simulink model "allmodes"  (Simulink 7.4)
settings: Solver=ode23tb  StartTime=0.0  StopTime=inf  MaxStep=1e-4  RelTol=1e-4
undefined symbols (not defined in the file): Ion, Lithium
libraries: powerlib x185, electricdrivelib x21, powerlib_extras x19, simulink x5
(part 1 of 7)
settings Model: RequirementInfo={} %GIDa_7aa36dfb_5f63_4103_a377_470aa43c19e1  Creator=SESHNUR  LastModifiedBy=Administrator

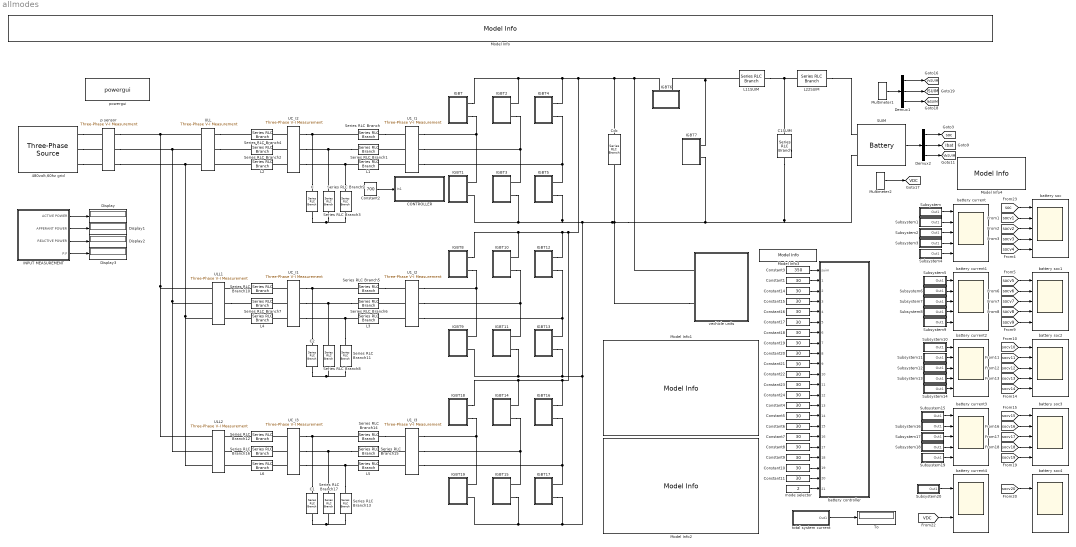
== system allmodes ==
  480volt,60hz grid : powerlib/Electrical Sources/Three-Phase Source  DialogController=POWERSYS.PowerSysDialog  SystemSampleTime=-1  Voltage=480  PhaseAngle=0  Frequency=60  InternalConnection=Yg  SpecifyImpedance=on  Resistance=0.8929  Inductance=16.58e-3  ShortCircuitLevel=50e6  BaseVoltage=400  XRratio=7
  C : powerlib/Elements/Series RLC Branch  DialogController=POWERSYS.PowerSysDialog  PhysicalDomain=powersysdomain  SubClassName=unknown  LeftPortType=p1  RightPortType=p1  LConnTagsString=__new0  RConnTagsString=__new0  BranchType=RC  Resistance=0.75  Inductance=1e-3  SetiL0=off  InitialCurrent=0  Capacitance=33e-6  Setx0=on  InitialVoltage=0  Measurements=Branch voltage and current
  C1 : powerlib/Elements/Series RLC Branch  DialogController=POWERSYS.PowerSysDialog  PhysicalDomain=powersysdomain  SubClassName=unknown  LeftPortType=p1  RightPortType=p1  LConnTagsString=__new0  RConnTagsString=__new0  BranchType=RC  Resistance=0.75  Inductance=1e-3  SetiL0=off  InitialCurrent=0  Capacitance=33e-6  Setx0=on  InitialVoltage=0  Measurements=Branch voltage and current
  C1SUIM : powerlib/Elements/Series RLC Branch  DialogController=POWERSYS.PowerSysDialog  PhysicalDomain=powersysdomain  SubClassName=unknown  LeftPortType=p1  RightPortType=p1  LConnTagsString=__new0  RConnTagsString=__new0  BranchType=C  Resistance=0.75  Inductance=1e-3  SetiL0=off  InitialCurrent=0  Capacitance=33e-6  Setx0=on  InitialVoltage=0  Measurements=Branch voltage and current
  C2 : powerlib/Elements/Series RLC Branch  DialogController=POWERSYS.PowerSysDialog  PhysicalDomain=powersysdomain  SubClassName=unknown  LeftPortType=p1  RightPortType=p1  LConnTagsString=__new0  RConnTagsString=__new0  BranchType=RC  Resistance=0.75  Inductance=1e-3  SetiL0=off  InitialCurrent=0  Capacitance=33e-6  Setx0=on  InitialVoltage=0  Measurements=Branch voltage and current
  CONTROLLER : Subsystem
  Cdc : powerlib/Elements/Series RLC Branch  DialogController=POWERSYS.PowerSysDialog  PhysicalDomain=powersysdomain  SubClassName=unknown  LeftPortType=p1  RightPortType=p1  LConnTagsString=__new0  RConnTagsString=__new0  BranchType=C  Resistance=0.002  Inductance=1e-3  SetiL0=off  InitialCurrent=0  Capacitance=0.5  Setx0=on  InitialVoltage=500  Measurements=Branch voltage and current
  Constant{1,4..11,14..24} (20 alike) : Constant  Value=30  OutDataType=fixdt(1, 16)  OutScaling=2^0
  Constant2 : Constant  Value=700  OutDataType=fixdt(1, 16)  OutScaling=2^0
  Constant3 : Constant  Value=350  OutDataType=fixdt(1, 16)  OutScaling=2^0
  Demux1 : Demux  Outputs=3
  Demux2 : Demux  Outputs=3
  Display{,1..3} (4 alike) : Display
  IGBT : Subsystem
  IGBT1 : Subsystem
  IGBT10 : Subsystem
  IGBT11 : Subsystem
  IGBT12 : Subsystem
  IGBT13 : Subsystem
  IGBT14 : Subsystem
  IGBT15 : Subsystem
  IGBT16 : Subsystem
  IGBT17 : Subsystem
  IGBT18 : Subsystem
  IGBT19 : Subsystem
  IGBT2 : Subsystem
  IGBT3 : Subsystem
  IGBT4 : Subsystem
  IGBT5 : Subsystem
  IGBT6 : Subsystem
  IGBT7 : Subsystem
  IGBT8 : Subsystem
  IGBT9 : Subsystem
  INPUT MEASUREMENT : Subsystem
  L1 : powerlib/Elements/Series RLC Branch  DialogController=POWERSYS.PowerSysDialog  PhysicalDomain=powersysdomain  SubClassName=unknown  LeftPortType=p1  RightPortType=p1  LConnTagsString=__new0  RConnTagsString=__new0  BranchType=RL  Resistance=1e-3  Inductance=5e-4  SetiL0=off  InitialCurrent=0  Capacitance=1e-6  Setx0=off  InitialVoltage=0  Measurements=Branch voltage
  L11SUIM : powerlib/Elements/Series RLC Branch  DialogController=POWERSYS.PowerSysDialog  PhysicalDomain=powersysdomain  SubClassName=unknown  LeftPortType=p1  RightPortType=p1  LConnTagsString=__new0  RConnTagsString=__new0  BranchType=RL  Resistance=1e-3  Inductance=0.0033  SetiL0=off  InitialCurrent=0  Capacitance=1e-6  Setx0=off  InitialVoltage=0  Measurements=Branch voltage and current
  L2 : powerlib/Elements/Series RLC Branch  DialogController=POWERSYS.PowerSysDialog  PhysicalDomain=powersysdomain  SubClassName=unknown  LeftPortType=p1  RightPortType=p1  LConnTagsString=__new0  RConnTagsString=__new0  BranchType=RL  Resistance=1e-3  Inductance=2.5e-4  SetiL0=off  InitialCurrent=0  Capacitance=1e-6  Setx0=off  InitialVoltage=0  Measurements=Branch voltage
  L22SUIM : powerlib/Elements/Series RLC Branch  DialogController=POWERSYS.PowerSysDialog  PhysicalDomain=powersysdomain  SubClassName=unknown  LeftPortType=p1  RightPortType=p1  LConnTagsString=__new0  RConnTagsString=__new0  BranchType=RL  Resistance=1e-3  Inductance=1.2e-4  SetiL0=off  InitialCurrent=0  Capacitance=1e-6  Setx0=off  InitialVoltage=0  Measurements=Branch current
  L3 : powerlib/Elements/Series RLC Branch  DialogController=POWERSYS.PowerSysDialog  PhysicalDomain=powersysdomain  SubClassName=unknown  LeftPortType=p1  RightPortType=p1  LConnTagsString=__new0  RConnTagsString=__new0  BranchType=RL  Resistance=1e-3  Inductance=5e-4  SetiL0=off  InitialCurrent=0  Capacitance=1e-6  Setx0=off  InitialVoltage=0  Measurements=Branch voltage
  L4 : powerlib/Elements/Series RLC Branch  DialogController=POWERSYS.PowerSysDialog  PhysicalDomain=powersysdomain  SubClassName=unknown  LeftPortType=p1  RightPortType=p1  LConnTagsString=__new0  RConnTagsString=__new0  BranchType=RL  Resistance=1e-3  Inductance=2.5e-4  SetiL0=off  InitialCurrent=0  Capacitance=1e-6  Setx0=off  InitialVoltage=0  Measurements=Branch voltage
  L5 : powerlib/Elements/Series RLC Branch  DialogController=POWERSYS.PowerSysDialog  PhysicalDomain=powersysdomain  SubClassName=unknown  LeftPortType=p1  RightPortType=p1  LConnTagsString=__new0  RConnTagsString=__new0  BranchType=RL  Resistance=1e-3  Inductance=5e-4  SetiL0=off  InitialCurrent=0  Capacitance=1e-6  Setx0=off  InitialVoltage=0  Measurements=Branch voltage
  L6 : powerlib/Elements/Series RLC Branch  DialogController=POWERSYS.PowerSysDialog  PhysicalDomain=powersysdomain  SubClassName=unknown  LeftPortType=p1  RightPortType=p1  LConnTagsString=__new0  RConnTagsString=__new0  BranchType=RL  Resistance=1e-3  Inductance=2.5e-4  SetiL0=off  InitialCurrent=0  Capacitance=1e-6  Setx0=off  InitialVoltage=0  Measurements=Branch voltage
  Model Info : simulink/Model-Wide Utilities/Model Info  SystemSampleTime=-1  InitialBlockCM=None  BlockCM=None  Frame=on  DisplayStringWithTags=BI-Directional/Centralized/fast charging system for plug-in and all electric vechicles with built-im energy storage interface and v2g and energy management system(EMS) with demand response capabilities  HorizontalTextAlignment=Center  LeftAlignmentValue=0.5  SourceBlockDiagram=allmodes  TagMaxNumber=20
  Model Info1 : simulink/Model-Wide Utilities/Model Info  SystemSampleTime=-1  InitialBlockCM=None  BlockCM=None  Frame=on  DisplayStringWithTags=|  HorizontalTextAlignment=Center  LeftAlignmentValue=0.5  SourceBlockDiagram=allmodes  TagMaxNumber=20
      | suim:
      |     ref-
      |      minimum current:-350
      |      maximum current:350
      | rating: 400v,350A
      |     charging time:
      |          i=(0.3c for trickle charge --350*0.3)
      |             (7c for fast charge --350*7)
      | -ve reference for discharge mode
      | +ve reference for charging mode
  Model Info2 : simulink/Model-Wide Utilities/Model Info  SystemSampleTime=-1  InitialBlockCM=None  BlockCM=None  Frame=on  DisplayStringWithTags=|  HorizontalTextAlignment=Center  LeftAlignmentValue=0.5  SourceBlockDiagram=allmodes  TagMaxNumber=20
      | vechicle::
      |     ref-
      |      minimum current:-30
      |      maximum current:30
      | rating: 200v,30A
      |     charging time:
      |          i=(0.3c for trickle charge --30*0.3)
      |             (7c for fast charge --30*7)
      | -ve reference for discharge mode
      | +ve reference for charging mode
  Model Info3 : simulink/Model-Wide Utilities/Model Info  SystemSampleTime=-1  InitialBlockCM=None  BlockCM=None  Frame=on  DisplayStringWithTags=reference  HorizontalTextAlignment=Left  LeftAlignmentValue=0.02  SourceBlockDiagram=allmodes  TagMaxNumber=20
  Model Info4 : simulink/Model-Wide Utilities/Model Info  SystemSampleTime=-1  InitialBlockCM=None  BlockCM=None  Frame=on  DisplayStringWithTags="yellow - reference pin-  actual"  HorizontalTextAlignment=Center  LeftAlignmentValue=0.5  SourceBlockDiagram=allmodes  TagMaxNumber=20
  Multimeter1 : powerlib/Measurements/Multimeter  SystemSampleTime=-1  PhasorSimulation=off  OutputType=Complex  sel=[3 118 119]  L=119  Gain=[1 1 1]  yselected={'Ub: C1SUIM','Ib: L11SUIM','Ib: L22SUIM'};  PSBOutputType=1  PSBequivalent=0  AxesSetting=[0,0.1,-100,100]  Display=0  SavedBlockNames=-11
  Multimeter2 : powerlib/Measurements/Multimeter  SystemSampleTime=-1  PhasorSimulation=off  OutputType=Complex  sel=45  L=119  Gain=1  yselected={'Ub: Cdc'};  PSBOutputType=1  PSBequivalent=0  AxesSetting=[0,0.1,-100,100]  Display=0  SavedBlockNames=-11
  SUIM : electricdrivelib/Extra Sources/Battery  DialogController=POWERSYS.PowerSysDialog  SystemSampleTime=-1  BatType=Lithium-Ion  ShowDetailedParameters=off  NomV=400  NomQ=350  SOC=50  PresetModel=on  MaxQ=350  FullV=465.5949  Dis_rate=152.1739  R=0.011429  Normal_OP=316.5217  expZone="[432.1543      17.19565]"  Dis_Char=off  current=[2500 1000]  Units=Ampere-hour  Batt_Tr=30
  Series RLC Branch{,1,5..6,14..15} (6 alike) : powerlib/Elements/Series RLC Branch  DialogController=POWERSYS.PowerSysDialog  PhysicalDomain=powersysdomain  SubClassName=unknown  LeftPortType=p1  RightPortType=p1  LConnTagsString=__new0  RConnTagsString=__new0  BranchType=RL  Resistance=1e-3  Inductance=5e-4  SetiL0=off  InitialCurrent=0  Capacitance=1e-6  Setx0=off  InitialVoltage=0  Measurements=None
  Series RLC Branch{2,4,7,10,12,16} (6 alike) : powerlib/Elements/Series RLC Branch  DialogController=POWERSYS.PowerSysDialog  PhysicalDomain=powersysdomain  SubClassName=unknown  LeftPortType=p1  RightPortType=p1  LConnTagsString=__new0  RConnTagsString=__new0  BranchType=RL  Resistance=1e-3  Inductance=2.5e-4  SetiL0=off  InitialCurrent=0  Capacitance=1e-6  Setx0=off  InitialVoltage=0  Measurements=None
  Series RLC Branch{3,8..9,11,13,17} (6 alike) : powerlib/Elements/Series RLC Branch  DialogController=POWERSYS.PowerSysDialog  PhysicalDomain=powersysdomain  SubClassName=unknown  LeftPortType=p1  RightPortType=p1  LConnTagsString=__new0  RConnTagsString=__new0  BranchType=RC  Resistance=0.75  Inductance=1e-3  SetiL0=off  InitialCurrent=0  Capacitance=33e-6  Setx0=on  InitialVoltage=0  Measurements=None
  Subsystem : Subsystem
  Subsystem1 : Subsystem
  Subsystem10 : Subsystem
  Subsystem11 : Subsystem
  Subsystem12 : Subsystem
  Subsystem13 : Subsystem
  Subsystem14 : Subsystem
  Subsystem15 : Subsystem
  Subsystem16 : Subsystem
  Subsystem17 : Subsystem
  Subsystem18 : Subsystem
  Subsystem19 : Subsystem
  Subsystem2 : Subsystem
  Subsystem20 : Subsystem
  Subsystem3 : Subsystem
  Subsystem4 : Subsystem
  Subsystem5 : Subsystem
  Subsystem6 : Subsystem
  Subsystem7 : Subsystem
  Subsystem8 : Subsystem
  Subsystem9 : Subsystem
  To : Display
  U1_I1 : powerlib/Measurements/Three-Phase V-I Measurement  DialogController=POWERSYS.PowerSysDialog  SystemSampleTime=-1  VoltageMeasurement=phase-to-phase  SetLabelV=on  LabelV=U1  Vpu=off  CurrentMeasurement=yes  SetLabelI=on  LabelI=I1  Ipu=off  Pbase=100e6  Vbase=500e3  OutputType=Complex  PhasorSimulation=off  PSBequivalent=0
  U1_I2 : powerlib/Measurements/Three-Phase V-I Measurement  DialogController=POWERSYS.PowerSysDialog  SystemSampleTime=-1  VoltageMeasurement=phase-to-phase  SetLabelV=on  LabelV=U11  Vpu=off  CurrentMeasurement=yes  SetLabelI=on  LabelI=I11  Ipu=off  Pbase=100e6  Vbase=500e3  OutputType=Complex  PhasorSimulation=off  PSBequivalent=0
  U1_I3 : powerlib/Measurements/Three-Phase V-I Measurement  DialogController=POWERSYS.PowerSysDialog  SystemSampleTime=-1  VoltageMeasurement=phase-to-phase  SetLabelV=on  LabelV=U111  Vpu=off  CurrentMeasurement=yes  SetLabelI=on  LabelI=I111  Ipu=off  Pbase=100e6  Vbase=500e3  OutputType=Complex  PhasorSimulation=off  PSBequivalent=0
  UC_I1 : powerlib/Measurements/Three-Phase V-I Measurement  DialogController=POWERSYS.PowerSysDialog  SystemSampleTime=-1  VoltageMeasurement=phase-to-ground  SetLabelV=on  LabelV=Uc1  Vpu=off  CurrentMeasurement=yes  SetLabelI=on  LabelI=I21  Ipu=off  Pbase=100e6  Vbase=500e3  OutputType=Complex  PhasorSimulation=off  PSBequivalent=0
  UC_I2 : powerlib/Measurements/Three-Phase V-I Measurement  DialogController=POWERSYS.PowerSysDialog  SystemSampleTime=-1  VoltageMeasurement=phase-to-ground  SetLabelV=on  LabelV=Uc  Vpu=off  CurrentMeasurement=yes  SetLabelI=on  LabelI=I2  Ipu=off  Pbase=100e6  Vbase=500e3  OutputType=Complex  PhasorSimulation=off  PSBequivalent=0
  UC_I3 : powerlib/Measurements/Three-Phase V-I Measurement  DialogController=POWERSYS.PowerSysDialog  SystemSampleTime=-1  VoltageMeasurement=phase-to-ground  SetLabelV=on  LabelV=Uc11  Vpu=off  CurrentMeasurement=yes  SetLabelI=on  LabelI=I211  Ipu=off  Pbase=100e6  Vbase=500e3  OutputType=Complex  PhasorSimulation=off  PSBequivalent=0
  ULL : powerlib/Measurements/Three-Phase V-I Measurement  DialogController=POWERSYS.PowerSysDialog  SystemSampleTime=-1  VoltageMeasurement=phase-to-ground  SetLabelV=on  LabelV=ULL  Vpu=off  CurrentMeasurement=yes  SetLabelI=on  LabelI=IL  Ipu=off  Pbase=100e6  Vbase=500e3  OutputType=Complex  PhasorSimulation=off  PSBequivalent=0
  ULL1 : powerlib/Measurements/Three-Phase V-I Measurement  DialogController=POWERSYS.PowerSysDialog  SystemSampleTime=-1  VoltageMeasurement=phase-to-ground  SetLabelV=on  LabelV=ULL1  Vpu=off  CurrentMeasurement=yes  SetLabelI=on  LabelI=IL1  Ipu=off  Pbase=100e6  Vbase=500e3  OutputType=Complex  PhasorSimulation=off  PSBequivalent=0
  ULL2 : powerlib/Measurements/Three-Phase V-I Measurement  DialogController=POWERSYS.PowerSysDialog  SystemSampleTime=-1  VoltageMeasurement=phase-to-ground  SetLabelV=on  LabelV=ULL11  Vpu=off  CurrentMeasurement=yes  SetLabelI=on  LabelI=IL11  Ipu=off  Pbase=100e6  Vbase=500e3  OutputType=Complex  PhasorSimulation=off  PSBequivalent=0
  "battery controller " : Subsystem
  battery current{,1..3} (4 alike) : Scope  NumInputPorts=5
      battery current settings: TimeRange=0.25  YMin=-250~202~195~0~0  YMax=2500~214~215~225~225  MaxDataPoints=50000  SampleInput=on  SampleTime=0.001
      battery current1 settings: TimeRange=0.25  YMin=0~0~0~0~0  YMax=225~225~225~225~225  MaxDataPoints=50000  SampleInput=on  SampleTime=0.001
      battery current2 settings: TimeRange=0.25  YMin=115~115~115~115~115  YMax=135~135~135~135~135  SaveName=ScopeData2  MaxDataPoints=50000  SampleInput=on  SampleTime=0.001
      battery current3 settings: TimeRange=0.25  YMin=189~189~189~189~189  YMax=196~196~196~196~196  SaveName=ScopeData4  MaxDataPoints=50000  SampleInput=on  SampleTime=0.001
  battery current4 : Scope  NumInputPorts=2
      settings: TimeRange=0.7000000000000001  YMin=0~706.475  YMax=210~706.75  SaveName=ScopeData5  MaxDataPoints=50000  SampleInput=on  SampleTime=0.001
  battery soc{,1..3} (4 alike) : Scope  NumInputPorts=5
      battery soc settings: TimeRange=0.25  YMin=50~10.487~50.487~50~50  YMax=50~10.4893~50.4893~50~50  SaveName=ScopeData3  MaxDataPoints=50000  SampleInput=on  SampleTime=0.001
      battery soc1 settings: TimeRange=0.25  YMin=2.00683~50.0074~50.0074~50.0074~50.0074  YMax=2.00707~50.0076~50.0076~50.0076~50.0076  SaveName=ScopeData6  MaxDataPoints=50000  SampleInput=on  SampleTime=0.001
      battery soc2 settings: TimeRange=0.25  YMin=0.0026805~0.0026805~0.0026805~0.0026805~0.0026805  YMax=0.0026845~0.0026845~0.0026845~0.0026845~0.0026845  SaveName=ScopeData8  MaxDataPoints=50000  SampleInput=on  SampleTime=0.001
      battery soc3 settings: TimeRange=0.25  YMin=0~0~0~0~0  YMax=130~130~130~130~130  SaveName=ScopeData9  MaxDataPoints=50000  SampleInput=on  SampleTime=0.001
  battery soc4 : Scope  NumInputPorts=2
      settings: TimeRange=0.25  YMin=47.5~-1  YMax=52.5~1  SaveName=ScopeData10  MaxDataPoints=50000  SampleInput=on  SampleTime=0.001
  mode selector : Constant  Value=2  OutDataType=fixdt(1, 16)  OutScaling=2^0
  p sensor : powerlib/Measurements/Three-Phase V-I Measurement  DialogController=POWERSYS.PowerSysDialog  SystemSampleTime=-1  VoltageMeasurement=phase-to-ground  SetLabelV=on  LabelV=VIN  Vpu=off  CurrentMeasurement=yes  SetLabelI=on  LabelI=IIN  Ipu=off  Pbase=100e6  Vbase=500e3  OutputType=Complex  PhasorSimulation=off  PSBequivalent=0
  powergui : powerlib/powergui  Priority=1  SystemSampleTime=-1  SimulationMode=Discrete  SampleTime=50e-6  frequency=60  SPID=off  DisableSnubberDevices=off  DisableRonSwitches=off  DisableVfSwitches=off  SwTol=0  Interpol=off  frequencyindice=60  echomessages=off  HookPort=off  DisplayEquations=off  FunctionMessages=off  EnableUseOfTLC=off  x0status=blocks  RestoreLinks=warning  Frange=[0:2:500]  Ylog=off  Xlog=on  ShowGrid=off  save=off  variable=ZData  ZoomFFT=on  StartTime=0.0  cycles=1  DisplayStyle=1  fundamental=60  FreqAxis=off  MaxFrequency=1000  frequencyindicesteady=1  RmsSteady=1  display=off  Ts=0  methode=off
  total system current : Subsystem
  vechicle units : Subsystem
  tag scope: ISUIM=global, IbSUIM=global, Ibat=global, VDC=global, VbSUIM=global, VcSUIM=global, soc=global
  wires:
  SUIM/1 -> Demux2/1
  Demux2/1 -> [soc]
  Demux2/2 -> [Ibat]
  Demux2/3 -> [VbSUIM]
  Multimeter1/1 -> Demux1/1
  INPUT MEASUREMENT/1(ACTIVE POWER) -> Display/1
  INPUT MEASUREMENT/2(APPERANT POWER) -> Display1/1
  INPUT MEASUREMENT/3(REACTIVE POWER) -> Display2/1
  INPUT MEASUREMENT/4(P.F) -> Display3/1
  Demux1/2 -> [ISUIM]
  Demux1/3 -> [IbSUIM]
  Demux1/1 -> [VcSUIM]
  Constant2/1 -> CONTROLLER/1(In1)
  Constant3/1 -> "battery controller "/1(suim)
  Constant1/1 -> "battery controller "/2(1)
  Constant14/1 -> "battery controller "/3(2)
  Constant15/1 -> "battery controller "/4(3)
  Constant16/1 -> "battery controller "/5(4)
  Constant17/1 -> "battery controller "/6(5)
  Constant18/1 -> "battery controller "/7(6)
  Constant19/1 -> "battery controller "/8(7)
  Constant20/1 -> "battery controller "/9(8)
  Constant21/1 -> "battery controller "/10(9)
  Constant22/1 -> "battery controller "/11(10)
  Constant23/1 -> "battery controller "/12(11)
  Constant24/1 -> "battery controller "/13(12)
  Constant4/1 -> "battery controller "/14(13)
  Constant5/1 -> "battery controller "/15(14)
  Constant6/1 -> "battery controller "/16(15)
  Constant7/1 -> "battery controller "/17(16)
  Constant8/1 -> "battery controller "/18(17)
  Constant9/1 -> "battery controller "/19(18)
  Constant10/1 -> "battery controller "/20(19)
  Constant11/1 -> "battery controller "/21(20)
  mode selector/1 -> "battery controller "/22(21)
  Multimeter2/1 -> [VDC]
  [VDC] -> battery current4/2
  Subsystem/1(Out1) -> battery current/1
  Subsystem1/1(Out1) -> battery current/2
  Subsystem2/1(Out1) -> battery current/3
  Subsystem3/1(Out1) -> battery current/4
  Subsystem4/1(Out1) -> battery current/5
  Subsystem5/1(Out1) -> battery current1/1
  Subsystem6/1(Out1) -> battery current1/2
  Subsystem7/1(Out1) -> battery current1/3
  Subsystem8/1(Out1) -> battery current1/4
  Subsystem9/1(Out1) -> battery current1/5
  Subsystem10/1(Out1) -> battery current2/1
  Subsystem11/1(Out1) -> battery current2/2
  Subsystem12/1(Out1) -> battery current2/3
  Subsystem13/1(Out1) -> battery current2/4
  Subsystem14/1(Out1) -> battery current2/5
  Subsystem15/1(Out1) -> battery current3/1
  Subsystem16/1(Out1) -> battery current3/2
  Subsystem17/1(Out1) -> battery current3/3
  Subsystem18/1(Out1) -> battery current3/4
  Subsystem19/1(Out1) -> battery current3/5
  Subsystem20/1(Out1) -> battery current4/1
  total system current/1(Out1) -> To/1
  [soc] -> battery soc/1
  [socv1] -> battery soc/2
  [socv2] -> battery soc/3
  [socv3] -> battery soc/4
  [socv4] -> battery soc/5
  [socv5] -> battery soc1/1
  [socv6] -> battery soc1/2
  [socv7] -> battery soc1/3
  [socv8] -> battery soc1/4
  [socv9] -> battery soc1/5
  [socv10] -> battery soc2/1
  [socv11] -> battery soc2/2
  [socv12] -> battery soc2/3
  [socv13] -> battery soc2/4
  [socv14] -> battery soc2/5
  [socv15] -> battery soc3/1
  [socv16] -> battery soc3/2
  [socv17] -> battery soc3/3
  [socv18] -> battery soc3/4
  [socv19] -> battery soc3/5
  [socv20] -> battery soc4/1
  connections:
  Series RLC Branch1/LConn1 -- Series RLC Branch3/LConn1 -- UC_I2/RConn2
  C/LConn1 -- UC_I2/RConn1 -- Series RLC Branch/LConn1
  Series RLC Branch9/LConn1 -- UC_I2/RConn3 -- L1/LConn1
  Series RLC Branch3/RConn1 -- C/RConn1 -- Series RLC Branch9/RConn1
  UC_I2/LConn3 -- L2/RConn1
  Series RLC Branch/RConn1 -- U1_I1/LConn1
  U1_I1/LConn3 -- L1/RConn1
  L2/LConn1 -- ULL/RConn3
  UC_I2/LConn2 -- Series RLC Branch2/RConn1
  UC_I2/LConn1 -- Series RLC Branch4/RConn1
  U1_I1/LConn2 -- Series RLC Branch1/RConn1
  ULL/RConn2 -- Series RLC Branch2/LConn1
  ULL/RConn1 -- Series RLC Branch4/LConn1
  IGBT/RConn2 -- IGBT1/RConn1 -- U1_I1/RConn1
  IGBT2/RConn2 -- IGBT3/RConn1 -- U1_I1/RConn2
  IGBT7/RConn1 -- IGBT6/RConn2 -- L11SUIM/LConn1
  IGBT4/RConn2 -- IGBT5/RConn1 -- U1_I1/RConn3
  L11SUIM/RConn1 -- L22SUIM/LConn1 -- C1SUIM/LConn1
  L22SUIM/RConn1 -- SUIM/LConn1
  Series RLC Branch6/LConn1 -- UC_I1/RConn2 -- Series RLC Branch8/LConn1
  C2/LConn1 -- Series RLC Branch5/LConn1 -- UC_I1/RConn1
  Series RLC Branch11/LConn1 -- L3/LConn1 -- UC_I1/RConn3
  Series RLC Branch8/RConn1 -- Series RLC Branch11/RConn1 -- C2/RConn1
  IGBT8/RConn2 -- U1_I2/RConn1 -- IGBT9/RConn1
  IGBT10/RConn2 -- U1_I2/RConn2 -- IGBT11/RConn1
  IGBT12/RConn2 -- U1_I2/RConn3 -- IGBT13/RConn1
  L4/LConn1 -- ULL1/RConn3
  ULL1/RConn1 -- Series RLC Branch10/LConn1
  U1_I2/LConn2 -- Series RLC Branch6/RConn1
  UC_I1/LConn3 -- L4/RConn1
  ULL1/RConn2 -- Series RLC Branch7/LConn1
  U1_I2/LConn3 -- L3/RConn1
  Series RLC Branch5/RConn1 -- U1_I2/LConn1
  UC_I1/LConn2 -- Series RLC Branch7/RConn1
  UC_I1/LConn1 -- Series RLC Branch10/RConn1
  480volt,60hz grid/RConn1 -- p sensor/LConn1
  480volt,60hz grid/RConn2 -- p sensor/LConn2
  480volt,60hz grid/RConn3 -- p sensor/LConn3
  p sensor/RConn3 -- ULL/LConn3 -- ULL1/LConn3 -- ULL2/LConn3
  p sensor/RConn2 -- ULL/LConn2 -- ULL1/LConn2 -- ULL2/LConn2
  p sensor/RConn1 -- ULL/LConn1 -- ULL1/LConn1 -- ULL2/LConn1
  Series RLC Branch15/LConn1 -- Series RLC Branch17/LConn1 -- UC_I3/RConn2
  C1/LConn1 -- UC_I3/RConn1 -- Series RLC Branch14/LConn1
  Series RLC Branch13/LConn1 -- UC_I3/RConn3 -- L5/LConn1
  Series RLC Branch17/RConn1 -- C1/RConn1 -- Series RLC Branch13/RConn1
  IGBT18/RConn2 -- IGBT19/RConn1 -- U1_I3/RConn1
  IGBT14/RConn2 -- IGBT15/RConn1 -- U1_I3/RConn2
  IGBT16/RConn2 -- IGBT17/RConn1 -- U1_I3/RConn3
  ULL2/RConn1 -- Series RLC Branch12/LConn1
  U1_I3/LConn2 -- Series RLC Branch15/RConn1
  ULL2/RConn2 -- Series RLC Branch16/LConn1
  UC_I3/LConn3 -- L6/RConn1
  L6/LConn1 -- ULL2/RConn3
  UC_I3/LConn2 -- Series RLC Branch16/RConn1
  U1_I3/LConn3 -- L5/RConn1
  UC_I3/LConn1 -- Series RLC Branch12/RConn1
  Series RLC Branch14/RConn1 -- U1_I3/LConn1
  vechicle units/LConn1 -- IGBT6/RConn1 -- IGBT12/RConn1 -- IGBT10/RConn1 -- IGBT8/RConn1 -- IGBT16/RConn1 -- IGBT18/RConn1 -- IGBT14/RConn1 -- IGBT4/RConn1 -- IGBT/RConn1 -- IGBT2/RConn1 -- Cdc/LConn1
  vechicle units/LConn2 -- IGBT17/RConn2 -- IGBT15/RConn2 -- IGBT19/RConn2 -- IGBT13/RConn2 -- IGBT9/RConn2 -- IGBT11/RConn2 -- IGBT5/RConn2 -- IGBT3/RConn2 -- IGBT1/RConn2 -- C1SUIM/RConn1 -- SUIM/LConn2 -- IGBT7/RConn2 -- Cdc/RConn1

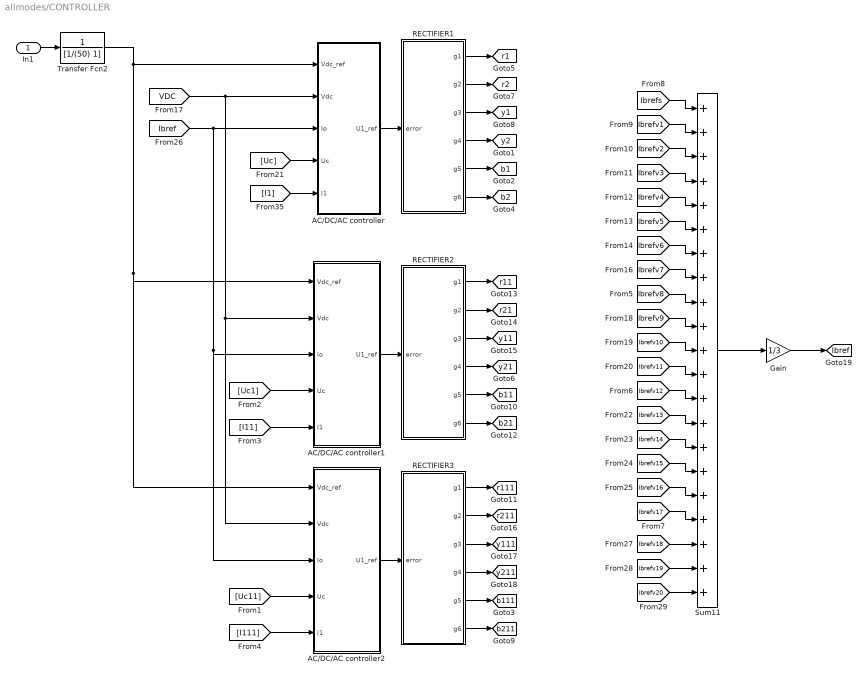
== system allmodes/CONTROLLER ==
  In1 : Inport
  AC/DC/AC controller : Subsystem
  AC/DC/AC controller1 : Subsystem
  AC/DC/AC controller2 : Subsystem
  Gain : Gain  Gain=1/3  ParameterDataType=fixdt(1, 16)  ParameterScaling=2^0  OutDataType=fixdt(1, 16)  OutScaling=2^0
  RECTIFIER1 : Subsystem  mask{fsw=5e3}
      mask prompts: fsw "switching frequency"
  RECTIFIER2 : Subsystem  mask{fsw=5e3}
      mask prompts: fsw "switching frequency"
  RECTIFIER3 : Subsystem  mask{fsw=5e3}
      mask prompts: fsw "switching frequency"
  Sum11 : Sum  Inputs=+++++++++++++++++++++  OutDataType=fixdt(1, 16)  OutScaling=2^0
  Transfer Fcn2 : TransferFcn  Numerator=1  Denominator=[1/(50) 1]
  tag scope: Ibref=global, b111=global, b11=global, b1=global, b211=global, b21=global, b2=global, r111=global, r11=global, r1=global, r211=global, r21=global, r2=global, y111=global, y11=global, y1=global, y211=global, y21=global, y2=global
  wires:
  RECTIFIER1/1(g1) -> [r1]
  RECTIFIER1/2(g2) -> [r2]
  RECTIFIER1/3(g3) -> [y1]
  RECTIFIER1/4(g4) -> [y2]
  RECTIFIER1/5(g5) -> [b1]
  RECTIFIER1/6(g6) -> [b2]
  RECTIFIER2/1(g1) -> [r11]
  RECTIFIER2/2(g2) -> [r21]
  RECTIFIER2/3(g3) -> [y11]
  RECTIFIER2/4(g4) -> [y21]
  RECTIFIER2/5(g5) -> [b11]
  RECTIFIER2/6(g6) -> [b21]
  [VDC] -> AC/DC/AC controller/2(Vdc), AC/DC/AC controller1/2(Vdc), AC/DC/AC controller2/2(Vdc)
  [Uc] -> AC/DC/AC controller/4(Uc)
  [I1] -> AC/DC/AC controller/5(I1)
  [Ibref] -> AC/DC/AC controller/3(Io), AC/DC/AC controller1/3(Io), AC/DC/AC controller2/3(Io)
  [Uc1] -> AC/DC/AC controller1/4(Uc)
  [I11] -> AC/DC/AC controller1/5(I1)
  AC/DC/AC controller/1(U1_ref) -> RECTIFIER1/1(error)
  AC/DC/AC controller1/1(U1_ref) -> RECTIFIER2/1(error)
  In1/1 -> Transfer Fcn2/1
  Transfer Fcn2/1 -> AC/DC/AC controller/1(Vdc_ref), AC/DC/AC controller1/1(Vdc_ref), AC/DC/AC controller2/1(Vdc_ref)
  RECTIFIER3/1(g1) -> [r111]
  RECTIFIER3/2(g2) -> [r211]
  RECTIFIER3/3(g3) -> [y111]
  RECTIFIER3/4(g4) -> [y211]
  RECTIFIER3/5(g5) -> [b111]
  RECTIFIER3/6(g6) -> [b211]
  [Uc11] -> AC/DC/AC controller2/4(Uc)
  [I111] -> AC/DC/AC controller2/5(I1)
  AC/DC/AC controller2/1(U1_ref) -> RECTIFIER3/1(error)
  [Ibrefs] -> Sum11/1
  [Ibrefv1] -> Sum11/2
  [Ibrefv2] -> Sum11/3
  [Ibrefv3] -> Sum11/4
  [Ibrefv4] -> Sum11/5
  [Ibrefv5] -> Sum11/6
  [Ibrefv6] -> Sum11/7
  [Ibrefv7] -> Sum11/8
  [Ibrefv8] -> Sum11/9
  [Ibrefv9] -> Sum11/10
  [Ibrefv10] -> Sum11/11
  [Ibrefv11] -> Sum11/12
  [Ibrefv12] -> Sum11/13
  [Ibrefv13] -> Sum11/14
  [Ibrefv14] -> Sum11/15
  [Ibrefv15] -> Sum11/16
  [Ibrefv16] -> Sum11/17
  [Ibrefv17] -> Sum11/18
  [Ibrefv18] -> Sum11/19
  [Ibrefv19] -> Sum11/20
  [Ibrefv20] -> Sum11/21
  Sum11/1 -> Gain/1
  Gain/1 -> [Ibref]

== system allmodes/IGBT ==
  IGBT/Diode : powerlib/Power Electronics/IGBT//Diode  DialogController=POWERSYS.PowerSysDialog  SystemSampleTime=-1  Ron=1e-3  Rs=1e5  Cs=inf  Measurements=off
  collector : PMIOPort  Port=1  Side=Right
  emitter : PMIOPort  Port=2  Side=Right
  wires:
  [r1] -> IGBT/Diode/1
  connections:
  collector/RConn1 -- IGBT/Diode/LConn1
  emitter/RConn1 -- IGBT/Diode/RConn1

== system allmodes/IGBT1 ==
  IGBT/Diode : powerlib/Power Electronics/IGBT//Diode  DialogController=POWERSYS.PowerSysDialog  SystemSampleTime=-1  Ron=1e-3  Rs=1e5  Cs=inf  Measurements=off
  collector : PMIOPort  Port=1  Side=Right
  emitter : PMIOPort  Port=2  Side=Right
  wires:
  [r2] -> IGBT/Diode/1
  connections:
  emitter/RConn1 -- IGBT/Diode/RConn1
  collector/RConn1 -- IGBT/Diode/LConn1

== system allmodes/IGBT10 ==
  IGBT/Diode : powerlib/Power Electronics/IGBT//Diode  DialogController=POWERSYS.PowerSysDialog  SystemSampleTime=-1  Ron=1e-3  Rs=1e5  Cs=inf  Measurements=off
  collector : PMIOPort  Port=1  Side=Right
  emitter : PMIOPort  Port=2  Side=Right
  wires:
  [y11] -> IGBT/Diode/1
  connections:
  collector/RConn1 -- IGBT/Diode/LConn1
  emitter/RConn1 -- IGBT/Diode/RConn1

== system allmodes/IGBT11 ==
  IGBT/Diode : powerlib/Power Electronics/IGBT//Diode  DialogController=POWERSYS.PowerSysDialog  SystemSampleTime=-1  Ron=1e-3  Rs=1e5  Cs=inf  Measurements=off
  collector : PMIOPort  Port=1  Side=Right
  emitter : PMIOPort  Port=2  Side=Right
  wires:
  [y21] -> IGBT/Diode/1
  connections:
  emitter/RConn1 -- IGBT/Diode/RConn1
  collector/RConn1 -- IGBT/Diode/LConn1

== system allmodes/IGBT12 ==
  IGBT/Diode : powerlib/Power Electronics/IGBT//Diode  DialogController=POWERSYS.PowerSysDialog  SystemSampleTime=-1  Ron=1e-3  Rs=1e5  Cs=inf  Measurements=off
  collector : PMIOPort  Port=1  Side=Right
  emitter : PMIOPort  Port=2  Side=Right
  wires:
  [b11] -> IGBT/Diode/1
  connections:
  emitter/RConn1 -- IGBT/Diode/RConn1
  collector/RConn1 -- IGBT/Diode/LConn1

== system allmodes/IGBT13 ==
  IGBT/Diode : powerlib/Power Electronics/IGBT//Diode  DialogController=POWERSYS.PowerSysDialog  SystemSampleTime=-1  Ron=1e-3  Rs=1e5  Cs=inf  Measurements=off
  collector : PMIOPort  Port=1  Side=Right
  emitter : PMIOPort  Port=2  Side=Right
  wires:
  [b21] -> IGBT/Diode/1
  connections:
  collector/RConn1 -- IGBT/Diode/LConn1
  emitter/RConn1 -- IGBT/Diode/RConn1

== system allmodes/IGBT14 ==
  IGBT/Diode : powerlib/Power Electronics/IGBT//Diode  DialogController=POWERSYS.PowerSysDialog  SystemSampleTime=-1  Ron=1e-3  Rs=1e5  Cs=inf  Measurements=off
  collector : PMIOPort  Port=1  Side=Right
  emitter : PMIOPort  Port=2  Side=Right
  wires:
  [y111] -> IGBT/Diode/1
  connections:
  emitter/RConn1 -- IGBT/Diode/RConn1
  collector/RConn1 -- IGBT/Diode/LConn1

== system allmodes/IGBT15 ==
  IGBT/Diode : powerlib/Power Electronics/IGBT//Diode  DialogController=POWERSYS.PowerSysDialog  SystemSampleTime=-1  Ron=1e-3  Rs=1e5  Cs=inf  Measurements=off
  collector : PMIOPort  Port=1  Side=Right
  emitter : PMIOPort  Port=2  Side=Right
  wires:
  [y211] -> IGBT/Diode/1
  connections:
  collector/RConn1 -- IGBT/Diode/LConn1
  emitter/RConn1 -- IGBT/Diode/RConn1

== system allmodes/IGBT16 ==
  IGBT/Diode : powerlib/Power Electronics/IGBT//Diode  DialogController=POWERSYS.PowerSysDialog  SystemSampleTime=-1  Ron=1e-3  Rs=1e5  Cs=inf  Measurements=off
  collector : PMIOPort  Port=1  Side=Right
  emitter : PMIOPort  Port=2  Side=Right
  wires:
  [b111] -> IGBT/Diode/1
  connections:
  collector/RConn1 -- IGBT/Diode/LConn1
  emitter/RConn1 -- IGBT/Diode/RConn1

== system allmodes/IGBT17 ==
  IGBT/Diode : powerlib/Power Electronics/IGBT//Diode  DialogController=POWERSYS.PowerSysDialog  SystemSampleTime=-1  Ron=1e-3  Rs=1e5  Cs=inf  Measurements=off
  collector : PMIOPort  Port=1  Side=Right
  emitter : PMIOPort  Port=2  Side=Right
  wires:
  [b211] -> IGBT/Diode/1
  connections:
  emitter/RConn1 -- IGBT/Diode/RConn1
  collector/RConn1 -- IGBT/Diode/LConn1

== system allmodes/IGBT18 ==
  IGBT/Diode : powerlib/Power Electronics/IGBT//Diode  DialogController=POWERSYS.PowerSysDialog  SystemSampleTime=-1  Ron=1e-3  Rs=1e5  Cs=inf  Measurements=off
  collector : PMIOPort  Port=1  Side=Right
  emitter : PMIOPort  Port=2  Side=Right
  wires:
  [r111] -> IGBT/Diode/1
  connections:
  collector/RConn1 -- IGBT/Diode/LConn1
  emitter/RConn1 -- IGBT/Diode/RConn1

== system allmodes/IGBT19 ==
  IGBT/Diode : powerlib/Power Electronics/IGBT//Diode  DialogController=POWERSYS.PowerSysDialog  SystemSampleTime=-1  Ron=1e-3  Rs=1e5  Cs=inf  Measurements=off
  collector : PMIOPort  Port=1  Side=Right
  emitter : PMIOPort  Port=2  Side=Right
  wires:
  [r211] -> IGBT/Diode/1
  connections:
  emitter/RConn1 -- IGBT/Diode/RConn1
  collector/RConn1 -- IGBT/Diode/LConn1

== system allmodes/IGBT2 ==
  IGBT/Diode : powerlib/Power Electronics/IGBT//Diode  DialogController=POWERSYS.PowerSysDialog  SystemSampleTime=-1  Ron=1e-3  Rs=1e5  Cs=inf  Measurements=off
  collector : PMIOPort  Port=1  Side=Right
  emitter : PMIOPort  Port=2  Side=Right
  wires:
  [y1] -> IGBT/Diode/1
  connections:
  emitter/RConn1 -- IGBT/Diode/RConn1
  collector/RConn1 -- IGBT/Diode/LConn1

== system allmodes/IGBT3 ==
  IGBT/Diode : powerlib/Power Electronics/IGBT//Diode  DialogController=POWERSYS.PowerSysDialog  SystemSampleTime=-1  Ron=1e-3  Rs=1e5  Cs=inf  Measurements=off
  collector : PMIOPort  Port=1  Side=Right
  emitter : PMIOPort  Port=2  Side=Right
  wires:
  [y2] -> IGBT/Diode/1
  connections:
  collector/RConn1 -- IGBT/Diode/LConn1
  emitter/RConn1 -- IGBT/Diode/RConn1

== system allmodes/IGBT4 ==
  IGBT/Diode : powerlib/Power Electronics/IGBT//Diode  DialogController=POWERSYS.PowerSysDialog  SystemSampleTime=-1  Ron=1e-3  Rs=1e5  Cs=inf  Measurements=off
  collector : PMIOPort  Port=1  Side=Right
  emitter : PMIOPort  Port=2  Side=Right
  wires:
  [b1] -> IGBT/Diode/1
  connections:
  collector/RConn1 -- IGBT/Diode/LConn1
  emitter/RConn1 -- IGBT/Diode/RConn1

== system allmodes/IGBT5 ==
  IGBT/Diode : powerlib/Power Electronics/IGBT//Diode  DialogController=POWERSYS.PowerSysDialog  SystemSampleTime=-1  Ron=1e-3  Rs=1e5  Cs=inf  Measurements=off
  collector : PMIOPort  Port=1  Side=Right
  emitter : PMIOPort  Port=2  Side=Right
  wires:
  [b2] -> IGBT/Diode/1
  connections:
  emitter/RConn1 -- IGBT/Diode/RConn1
  collector/RConn1 -- IGBT/Diode/LConn1

== system allmodes/IGBT6 ==
  IGBT/Diode : powerlib/Power Electronics/IGBT//Diode  DialogController=POWERSYS.PowerSysDialog  SystemSampleTime=-1  Ron=1e-3  Rs=1e5  Cs=inf  Measurements=off
  collector : PMIOPort  Port=1  Side=Right
  emitter : PMIOPort  Port=2  Side=Right
  wires:
  [buck] -> IGBT/Diode/1
  connections:
  emitter/RConn1 -- IGBT/Diode/RConn1
  collector/RConn1 -- IGBT/Diode/LConn1

== system allmodes/IGBT7 ==
  IGBT/Diode : powerlib/Power Electronics/IGBT//Diode  DialogController=POWERSYS.PowerSysDialog  SystemSampleTime=-1  Ron=1e-3  Rs=1e5  Cs=inf  Measurements=off
  collector : PMIOPort  Port=1  Side=Right
  emitter : PMIOPort  Port=2  Side=Right
  wires:
  [boost] -> IGBT/Diode/1
  connections:
  collector/RConn1 -- IGBT/Diode/LConn1
  emitter/RConn1 -- IGBT/Diode/RConn1

== system allmodes/IGBT8 ==
  IGBT/Diode : powerlib/Power Electronics/IGBT//Diode  DialogController=POWERSYS.PowerSysDialog  SystemSampleTime=-1  Ron=1e-3  Rs=1e5  Cs=inf  Measurements=off
  collector : PMIOPort  Port=1  Side=Right
  emitter : PMIOPort  Port=2  Side=Right
  wires:
  [r11] -> IGBT/Diode/1
  connections:
  emitter/RConn1 -- IGBT/Diode/RConn1
  collector/RConn1 -- IGBT/Diode/LConn1

== system allmodes/IGBT9 ==
  IGBT/Diode : powerlib/Power Electronics/IGBT//Diode  DialogController=POWERSYS.PowerSysDialog  SystemSampleTime=-1  Ron=1e-3  Rs=1e5  Cs=inf  Measurements=off
  collector : PMIOPort  Port=1  Side=Right
  emitter : PMIOPort  Port=2  Side=Right
  wires:
  [r21] -> IGBT/Diode/1
  connections:
  collector/RConn1 -- IGBT/Diode/LConn1
  emitter/RConn1 -- IGBT/Diode/RConn1

== system allmodes/INPUT MEASUREMENT ==
  3-phase  Instantaneous  Active & Reactive Power : powerlib_extras/Measurements/3-phase  Instantaneous  Active & Reactive Power  DialogController=POWERSYS.PowerSysDialog  SystemSampleTime=-1
  Add : Sum  OutDataType=fixdt(1, 16)  OutScaling=2^-10
  Demux : Demux  Outputs=2
  Divide : Product  Inputs=*/  OutDataType=fixdt(1, 16)  OutScaling=2^-10
  Fcn : Fcn  Expr=u(1)*u(1)
  Fcn1 : Fcn  Expr=u(1)*u(1)
  Math Function : Math  Operator=sqrt  OutDataType=fixdt(1, 16)  OutScaling=2^0  SaturateOnIntegerOverflow=on
  ACTIVE POWER : Outport
  APPERANT POWER : Outport  Port=2
  REACTIVE POWER : Outport  Port=3
  P.F : Outport  Port=4
  wires:
  Add/1 -> Math Function/1
  Fcn1/1 -> Add/2
  Fcn/1 -> Add/1
  Demux/2 -> Fcn1/1, REACTIVE POWER/1
  Demux/1 -> Fcn/1, Divide/1, ACTIVE POWER/1
  3-phase  Instantaneous  Active & Reactive Power/1 -> Demux/1
  Math Function/1 -> Divide/2, APPERANT POWER/1
  [VIN] -> 3-phase  Instantaneous  Active & Reactive Power/1
  [IIN] -> 3-phase  Instantaneous  Active & Reactive Power/2
  Divide/1 -> P.F/1

== system allmodes/Subsystem ==
  Mux : Mux  Inputs=2
  Out1 : Outport
  wires:
  [Ibrefs] -> Mux/1
  [ISUIM] -> Mux/2
  Mux/1 -> Out1/1

== system allmodes/Subsystem1 ==
  Mux : Mux  Inputs=2
  Out1 : Outport
  wires:
  [Ibrefv1] -> Mux/1
  [ISUIMv1] -> Mux/2
  Mux/1 -> Out1/1

== system allmodes/Subsystem10 ==
  Mux : Mux  Inputs=2
  Out1 : Outport
  wires:
  Mux/1 -> Out1/1
  [ISUIMv10] -> Mux/2
  [Ibrefv10] -> Mux/1

== system allmodes/Subsystem11 ==
  Mux : Mux  Inputs=2
  Out1 : Outport
  wires:
  [Ibrefv11] -> Mux/1
  [ISUIMv11] -> Mux/2
  Mux/1 -> Out1/1

== system allmodes/Subsystem12 ==
  Mux : Mux  Inputs=2
  Out1 : Outport
  wires:
  Mux/1 -> Out1/1
  [ISUIMv12] -> Mux/2
  [Ibrefv12] -> Mux/1

== system allmodes/Subsystem13 ==
  Mux : Mux  Inputs=2
  Out1 : Outport
  wires:
  [Ibrefv13] -> Mux/1
  [ISUIMv13] -> Mux/2
  Mux/1 -> Out1/1

== system allmodes/Subsystem14 ==
  Mux : Mux  Inputs=2
  Out1 : Outport
  wires:
  Mux/1 -> Out1/1
  [ISUIMv14] -> Mux/2
  [Ibrefv14] -> Mux/1

== system allmodes/Subsystem15 ==
  Mux : Mux  Inputs=2
  Out1 : Outport
  wires:
  [Ibrefv15] -> Mux/1
  [ISUIMv15] -> Mux/2
  Mux/1 -> Out1/1

== system allmodes/Subsystem16 ==
  Mux : Mux  Inputs=2
  Out1 : Outport
  wires:
  Mux/1 -> Out1/1
  [ISUIMv16] -> Mux/2
  [Ibrefv16] -> Mux/1

== system allmodes/Subsystem17 ==
  Mux : Mux  Inputs=2
  Out1 : Outport
  wires:
  [Ibrefv17] -> Mux/1
  [ISUIMv17] -> Mux/2
  Mux/1 -> Out1/1

== system allmodes/Subsystem18 ==
  Mux : Mux  Inputs=2
  Out1 : Outport
  wires:
  Mux/1 -> Out1/1
  [ISUIMv18] -> Mux/2
  [Ibrefv18] -> Mux/1

== system allmodes/Subsystem19 ==
  Mux : Mux  Inputs=2
  Out1 : Outport
  wires:
  [Ibrefv19] -> Mux/1
  [ISUIMv19] -> Mux/2
  Mux/1 -> Out1/1

== system allmodes/Subsystem2 ==
  Mux : Mux  Inputs=2
  Out1 : Outport
  wires:
  Mux/1 -> Out1/1
  [ISUIMv2] -> Mux/2
  [Ibrefv2] -> Mux/1

== system allmodes/Subsystem20 ==
  Mux : Mux  Inputs=2
  Out1 : Outport
  wires:
  Mux/1 -> Out1/1
  [ISUIMv20] -> Mux/2
  [Ibrefv20] -> Mux/1

== system allmodes/Subsystem3 ==
  Mux : Mux  Inputs=2
  Out1 : Outport
  wires:
  [Ibrefv3] -> Mux/1
  [ISUIMv3] -> Mux/2
  Mux/1 -> Out1/1

== system allmodes/Subsystem4 ==
  Mux : Mux  Inputs=2
  Out1 : Outport
  wires:
  Mux/1 -> Out1/1
  [ISUIMv4] -> Mux/2
  [Ibrefv4] -> Mux/1

== system allmodes/Subsystem5 ==
  Mux : Mux  Inputs=2
  Out1 : Outport
  wires:
  [Ibrefv5] -> Mux/1
  [ISUIMv5] -> Mux/2
  Mux/1 -> Out1/1

== system allmodes/Subsystem6 ==
  Mux : Mux  Inputs=2
  Out1 : Outport
  wires:
  Mux/1 -> Out1/1
  [ISUIMv6] -> Mux/2
  [Ibrefv6] -> Mux/1

== system allmodes/Subsystem7 ==
  Mux : Mux  Inputs=2
  Out1 : Outport
  wires:
  [Ibrefv7] -> Mux/1
  [ISUIMv7] -> Mux/2
  Mux/1 -> Out1/1

== system allmodes/Subsystem8 ==
  Mux : Mux  Inputs=2
  Out1 : Outport
  wires:
  Mux/1 -> Out1/1
  [ISUIMv8] -> Mux/2
  [Ibrefv8] -> Mux/1

== system allmodes/Subsystem9 ==
  Mux : Mux  Inputs=2
  Out1 : Outport
  wires:
  [Ibrefv9] -> Mux/1
  [ISUIMv9] -> Mux/2
  Mux/1 -> Out1/1

== system allmodes/battery controller  ==
  suim : Inport
  1 : Inport  Port=2
  2 : Inport  Port=3
  3 : Inport  Port=4
  4 : Inport  Port=5
  5 : Inport  Port=6
  6 : Inport  Port=7
  7 : Inport  Port=8
  8 : Inport  Port=9
  9 : Inport  Port=10
  10 : Inport  Port=11
  11 : Inport  Port=12
  12 : Inport  Port=13
  13 : Inport  Port=14
  14 : Inport  Port=15
  15 : Inport  Port=16
  16 : Inport  Port=17
  17 : Inport  Port=18
  18 : Inport  Port=19
  19 : Inport  Port=20
  20 : Inport  Port=21
  21 : Inport  Port=22
  SUIM1 : Subsystem
  mode selector : Subsystem
  v1 : Subsystem
  v10 : Subsystem
  v11 : Subsystem
  v12 : Subsystem
  v13 : Subsystem
  v14 : Subsystem
  v15 : Subsystem
  v16 : Subsystem
  v17 : Subsystem
  v18 : Subsystem
  v19 : Subsystem
  v2 : Subsystem
  v20 : Subsystem
  v3 : Subsystem
  v4 : Subsystem
  v5 : Subsystem
  v6 : Subsystem
  v7 : Subsystem
  v8 : Subsystem
  v9 : Subsystem
  wires:
  suim/1 -> SUIM1/1(Ibref-SUIM)
  11/1 -> v11/1(Ibref-SUIM)
  1/1 -> v1/1(Ibref-SUIM)
  12/1 -> v12/1(Ibref-SUIM)
  2/1 -> v2/1(Ibref-v2)
  13/1 -> v13/1(Ibref-SUIM)
  3/1 -> v3/1(Ibref-v2)
  14/1 -> v14/1(Ibref-SUIM)
  4/1 -> v4/1(Ibref-v2)
  15/1 -> v15/1(Ibref-SUIM)
  5/1 -> v5/1(Ibref-v2)
  16/1 -> v16/1(Ibref-SUIM)
  6/1 -> v6/1(Ibref-v2)
  17/1 -> v17/1(Ibref-SUIM)
  7/1 -> v7/1(Ibref-v2)
  18/1 -> v18/1(Ibref-SUIM)
  8/1 -> v8/1(Ibref-v2)
  19/1 -> v19/1(Ibref-SUIM)
  9/1 -> v9/1(Ibref-v2)
  20/1 -> v20/1(Ibref-v2)
  10/1 -> v10/1(Ibref-SUIM)
  21/1 -> mode selector/1(In1)

== system allmodes/total system current ==
  Sum11 : Sum  Inputs=+++++++++++++++++++++  OutDataType=fixdt(1, 16)  OutScaling=2^0
  Out1 : Outport
  wires:
  [ISUIM] -> Sum11/1
  [ISUIMv1] -> Sum11/2
  [ISUIMv2] -> Sum11/3
  [ISUIMv3] -> Sum11/4
  [ISUIMv4] -> Sum11/5
  [ISUIMv5] -> Sum11/6
  [ISUIMv6] -> Sum11/7
  [ISUIMv7] -> Sum11/8
  [ISUIMv8] -> Sum11/9
  [ISUIMv9] -> Sum11/10
  [ISUIMv10] -> Sum11/11
  [ISUIMv11] -> Sum11/12
  [ISUIMv12] -> Sum11/13
  [ISUIMv13] -> Sum11/14
  [ISUIMv14] -> Sum11/15
  [ISUIMv15] -> Sum11/16
  [ISUIMv16] -> Sum11/17
  [ISUIMv17] -> Sum11/18
  [ISUIMv18] -> Sum11/19
  [ISUIMv19] -> Sum11/20
  [ISUIMv20] -> Sum11/21
  Sum11/1 -> Out1/1

== system allmodes/vechicle units ==
  vechicle-1 : Subsystem
  vechicle-10 : Subsystem
  vechicle-11 : Subsystem
  vechicle-12 : Subsystem
  vechicle-13 : Subsystem
  vechicle-14 : Subsystem
  vechicle-15 : Subsystem
  vechicle-16 : Subsystem
  vechicle-17 : Subsystem
  vechicle-18 : Subsystem
  vechicle-19 : Subsystem
  vechicle-2 : Subsystem
  vechicle-20 : Subsystem
  vechicle-3 : Subsystem
  vechicle-4 : Subsystem
  vechicle-5 : Subsystem
  vechicle-6 : Subsystem
  vechicle-7 : Subsystem
  vechicle-8 : Subsystem
  vechicle-9 : Subsystem
  +ve : PMIOPort  Port=1  Side=Left
  -ve : PMIOPort  Port=2  Side=Left
  connections:
  +ve/RConn1 -- vechicle-1/LConn1 -- vechicle-2/LConn1 -- vechicle-3/LConn1 -- vechicle-4/LConn1 -- vechicle-5/LConn1 -- vechicle-6/LConn1 -- vechicle-7/LConn1 -- vechicle-8/LConn1 -- vechicle-9/LConn1 -- vechicle-10/LConn1 -- vechicle-11/LConn1 -- vechicle-12/LConn1 -- vechicle-13/LConn1 -- vechicle-14/LConn1 -- vechicle-15/LConn1 -- vechicle-16/LConn1 -- vechicle-17/LConn1 -- vechicle-18/LConn1 -- vechicle-19/LConn1 -- vechicle-20/LConn1
  -ve/RConn1 -- vechicle-1/LConn2 -- vechicle-2/LConn2 -- vechicle-3/LConn2 -- vechicle-5/LConn2 -- vechicle-4/LConn2 -- vechicle-6/LConn2 -- vechicle-7/LConn2 -- vechicle-8/LConn2 -- vechicle-9/LConn2 -- vechicle-10/LConn2 -- vechicle-11/LConn2 -- vechicle-12/LConn2 -- vechicle-13/LConn2 -- vechicle-14/LConn2 -- vechicle-15/LConn2 -- vechicle-16/LConn2 -- vechicle-17/LConn2 -- vechicle-18/LConn2 -- vechicle-19/LConn2 -- vechicle-20/LConn2

== system allmodes/CONTROLLER/AC/DC/AC controller ==
  Vdc_ref : Inport
  Vdc : Inport  Port=2
  Io : Inport  Port=3
  Uc : Inport  Port=4
  I1 : Inport  Port=5
  I-D REF : Subsystem
  abc-dq : Subsystem
  abc-dq2 : Subsystem
  abc-dq4 : Subsystem
  current  controller : Subsystem
  U1_ref : Outport
  wires:
  current  controller/1(Vi_dq_ref) -> abc-dq4/1(In1)
  Vdc/1 -> I-D REF/2(Vdc), current  controller/4(Vdc)
  Io/1 -> I-D REF/3(Io)
  Uc/1 -> abc-dq/1(In1)
  I1/1 -> abc-dq2/1(In1)
  abc-dq4/1(q) -> U1_ref/1
  Vdc_ref/1 -> I-D REF/1(Vdc_ref)
  I-D REF/1(Id_ref) -> current  controller/1(Id_ref)
  abc-dq2/1(d) -> current  controller/2(Idq)
  abc-dq/1(d) -> current  controller/3(Vc_dq)

== system allmodes/CONTROLLER/AC/DC/AC controller1 ==
  Vdc_ref : Inport
  Vdc : Inport  Port=2
  Io : Inport  Port=3
  Uc : Inport  Port=4
  I1 : Inport  Port=5
  I-D REF : Subsystem
  abc-dq : Subsystem
  abc-dq2 : Subsystem
  abc-dq4 : Subsystem
  current  controller : Subsystem
  U1_ref : Outport
  wires:
  abc-dq/1(d) -> current  controller/3(Vc_dq)
  abc-dq2/1(d) -> current  controller/2(Idq)
  I-D REF/1(Id_ref) -> current  controller/1(Id_ref)
  Vdc_ref/1 -> I-D REF/1(Vdc_ref)
  abc-dq4/1(q) -> U1_ref/1
  I1/1 -> abc-dq2/1(In1)
  Uc/1 -> abc-dq/1(In1)
  Io/1 -> I-D REF/3(Io)
  Vdc/1 -> I-D REF/2(Vdc), current  controller/4(Vdc)
  current  controller/1(Vi_dq_ref) -> abc-dq4/1(In1)

== system allmodes/CONTROLLER/AC/DC/AC controller2 ==
  Vdc_ref : Inport
  Vdc : Inport  Port=2
  Io : Inport  Port=3
  Uc : Inport  Port=4
  I1 : Inport  Port=5
  I-D REF : Subsystem
  abc-dq : Subsystem
  abc-dq2 : Subsystem
  abc-dq4 : Subsystem
  current  controller : Subsystem
  U1_ref : Outport
  wires:
  current  controller/1(Vi_dq_ref) -> abc-dq4/1(In1)
  Vdc/1 -> I-D REF/2(Vdc), current  controller/4(Vdc)
  Io/1 -> I-D REF/3(Io)
  Uc/1 -> abc-dq/1(In1)
  I1/1 -> abc-dq2/1(In1)
  abc-dq4/1(q) -> U1_ref/1
  Vdc_ref/1 -> I-D REF/1(Vdc_ref)
  I-D REF/1(Id_ref) -> current  controller/1(Id_ref)
  abc-dq2/1(d) -> current  controller/2(Idq)
  abc-dq/1(d) -> current  controller/3(Vc_dq)

== system allmodes/CONTROLLER/RECTIFIER1 ==
  error : Inport  OutDataType=fixdt(1, 16)  OutScaling=2^0
  Data Type Conversion : DataTypeConversion  OutDataType=fixdt(1, 16)  OutScaling=2^0
  Data Type Conversion1 : DataTypeConversion  OutDataType=fixdt(1, 16)  OutScaling=2^0
  Demux : Demux  Outputs=3
  Demux1 : Demux  Outputs=3
  Relational Operator : RelationalOperator  Operator=>  LogicOutDataTypeMode=boolean  LogicDataType=fixdt(0, 8)  OutDataTypeStr=boolean
  Relational Operator1 : RelationalOperator  Operator=<  LogicOutDataTypeMode=boolean  LogicDataType=fixdt(0, 8)  OutDataTypeStr=boolean
  triangular wave gen1 : Subsystem  mask{fsw=fsw, mag=1}
      mask prompts: fsw "switching frequency"; mag "carrier magnitude"
  g1 : Outport
  g2 : Outport  Port=2
  g3 : Outport  Port=3
  g4 : Outport  Port=4
  g5 : Outport  Port=5
  g6 : Outport  Port=6
  wires:
  triangular wave gen1/1(tri_out) -> Relational Operator/2, Relational Operator1/2
  Relational Operator1/1 -> Data Type Conversion/1
  Relational Operator/1 -> Data Type Conversion1/1
  Demux1/1 -> g1/1
  Demux/1 -> g2/1
  Demux1/2 -> g3/1
  Demux/2 -> g4/1
  Demux1/3 -> g5/1
  Demux/3 -> g6/1
  Data Type Conversion/1 -> Demux/1
  Data Type Conversion1/1 -> Demux1/1
  error/1 -> Relational Operator/1, Relational Operator1/1

== system allmodes/CONTROLLER/RECTIFIER2 ==
  error : Inport  OutDataType=fixdt(1, 16)  OutScaling=2^0
  Data Type Conversion : DataTypeConversion  OutDataType=fixdt(1, 16)  OutScaling=2^0
  Data Type Conversion1 : DataTypeConversion  OutDataType=fixdt(1, 16)  OutScaling=2^0
  Demux : Demux  Outputs=3
  Demux1 : Demux  Outputs=3
  Relational Operator : RelationalOperator  Operator=>  LogicOutDataTypeMode=boolean  LogicDataType=fixdt(0, 8)  OutDataTypeStr=boolean
  Relational Operator1 : RelationalOperator  Operator=<  LogicOutDataTypeMode=boolean  LogicDataType=fixdt(0, 8)  OutDataTypeStr=boolean
  triangular wave gen1 : Subsystem  mask{fsw=fsw, mag=1}
      mask prompts: fsw "switching frequency"; mag "carrier magnitude"
  g1 : Outport
  g2 : Outport  Port=2
  g3 : Outport  Port=3
  g4 : Outport  Port=4
  g5 : Outport  Port=5
  g6 : Outport  Port=6
  wires:
  error/1 -> Relational Operator1/1, Relational Operator/1
  Data Type Conversion1/1 -> Demux1/1
  Data Type Conversion/1 -> Demux/1
  Demux/3 -> g6/1
  Demux1/3 -> g5/1
  Demux/2 -> g4/1
  Demux1/2 -> g3/1
  Demux/1 -> g2/1
  Demux1/1 -> g1/1
  Relational Operator/1 -> Data Type Conversion1/1
  Relational Operator1/1 -> Data Type Conversion/1
  triangular wave gen1/1(tri_out) -> Relational Operator1/2, Relational Operator/2

== system allmodes/CONTROLLER/RECTIFIER3 ==
  error : Inport  OutDataType=fixdt(1, 16)  OutScaling=2^0
  Data Type Conversion : DataTypeConversion  OutDataType=fixdt(1, 16)  OutScaling=2^0
  Data Type Conversion1 : DataTypeConversion  OutDataType=fixdt(1, 16)  OutScaling=2^0
  Demux : Demux  Outputs=3
  Demux1 : Demux  Outputs=3
  Relational Operator : RelationalOperator  Operator=>  LogicOutDataTypeMode=boolean  LogicDataType=fixdt(0, 8)  OutDataTypeStr=boolean
  Relational Operator1 : RelationalOperator  Operator=<  LogicOutDataTypeMode=boolean  LogicDataType=fixdt(0, 8)  OutDataTypeStr=boolean
  triangular wave gen1 : Subsystem  mask{fsw=fsw, mag=1}
      mask prompts: fsw "switching frequency"; mag "carrier magnitude"
  g1 : Outport
  g2 : Outport  Port=2
  g3 : Outport  Port=3
  g4 : Outport  Port=4
  g5 : Outport  Port=5
  g6 : Outport  Port=6
  wires:
  triangular wave gen1/1(tri_out) -> Relational Operator/2, Relational Operator1/2
  Relational Operator1/1 -> Data Type Conversion/1
  Relational Operator/1 -> Data Type Conversion1/1
  Demux1/1 -> g1/1
  Demux/1 -> g2/1
  Demux1/2 -> g3/1
  Demux/2 -> g4/1
  Demux1/3 -> g5/1
  Demux/3 -> g6/1
  Data Type Conversion/1 -> Demux/1
  Data Type Conversion1/1 -> Demux1/1
  error/1 -> Relational Operator/1, Relational Operator1/1
